simulink model "ReducedOrderStateSpace"  (R2015b)
settings: Solver=VariableStepAuto  StartTime=0.0  StopTime=10.0  RelTol=1e-3
undefined symbols (not defined in the file): c_drag_pro, J_pro, Kt, Kv, R, T_L, Vin
settings Model: Creator=Morten  LastModifiedBy=Morten

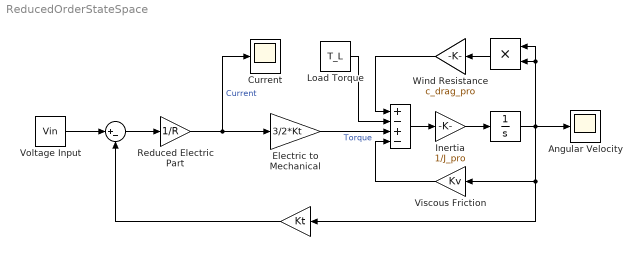
== system ReducedOrderStateSpace ==
  " " : Product
  "  " : Sum  Inputs=|+-
  "    " : Sum  Inputs=+-+-
  "                            " : Gain  Gain=Kt
  "                                     " : Integrator
  Angular Velocity : Scope
  Current : Scope
  Electric to Mechanical : Gain  Gain=3/2*Kt
  Inertia : Gain  Gain=1/J_pro
  Load Torque : Constant  Value=T_L
  Reduced Electric Part : Gain  Gain=1/R
  Viscous Friction : Gain  Gain=Kv
  Voltage Input : Constant  Value=Vin
  Wind Resistance : Gain  Gain=c_drag_pro
  wires:
  " "/1 -> Wind Resistance/1
  "    "/1 -> Inertia/1
  Reduced Electric Part/1 -> Current/1, Electric to Mechanical/1  "Current"
  "                            "/1 -> "  "/2
  Inertia/1 -> "                                     "/1
  "  "/1 -> Reduced Electric Part/1
  Voltage Input/1 -> "  "/1
  "                                     "/1 -> " "/1, " "/2, Angular Velocity/1, "                            "/1, Viscous Friction/1
  Wind Resistance/1 -> "    "/1
  Load Torque/1 -> "    "/2
  Electric to Mechanical/1 -> "    "/3  "Torque"
  Viscous Friction/1 -> "    "/4
